simulink library "rst_controller_lib"  (Simulink 4.00)
undefined symbols (not defined in the file or in its folder): motor_1, parameters, rst_controller_sysCallback
settings Model: LastModifiedBy=Nick Donaldson

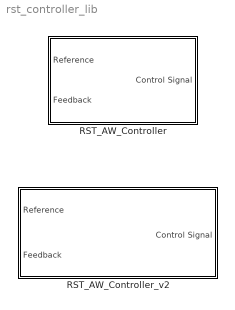
== system rst_controller_lib ==
  RST_AW_Controller : Subsystem  mask(RST Controller Design){Get_Controller_file=on, controll_fname='GLA_BEN_04_02_23_motorSim_1', R=motor_1.Controller_Design_1.rst_ctrl.R, S=motor_1.Controller_Design_1.rst_ctrl.S, T=motor_1.Controller_Design_1.rst_ctrl.T, Aaw=motor_1.Controller_Design_1.rst_ctrl.Aaw, Aaw_R=motor_1.Controller_Design_1.rst_ctrl.Aaw_R, out_limit=parameters.motor_controller.saturation_limit, sT=parameters.motor_controller.sample_time}
      mask prompts: Get_Controller_file "Get Controller from File"; controll_fname "Controller file name"; Aaw_R "Aaw - R"; out_limit "Output limitations"; sT "Sample time"
      mask help: Design of a controller that takes the form R*u = T*ref - S*output
      mask init:
      | if Get_Controller_file
      |    ctr_data = load(['Controllers\', controll_fname]);
      |    R = ctr_data.controllerData.rst.rst_ctrl.R;
      |    S = ctr_data.controllerData.rst.rst_ctrl.S;
      |    T = ctr_data.controllerData.rst.rst_ctrl.T;
      |    Aaw = ctr_data.controllerData.rst.rst_ctrl.Aaw;
      |    Aaw_R = ctr_data.controllerData.rst.rst_ctrl.Aaw_R;
      | end
      settings: RTWFcnNameOpts=Auto  RTWFileNameOpts=Auto
      mask CallbackString:
      | mv = get_param(gcb, 'MaskValues');
      |  if strcmp(mv{1}, 'on') a = 'on'; b = 'off';
      |  else a = 'off'; b = 'on';
      |  end;
      |  me = get_param(gcb, 'MaskEnables');
      |  me{2} = a;
      |  me{3} = b;
      |  me{4} = b;
      |  me{5} = b;
      |  me{6} = b;
      |  me{7} = b;
      |  set_param(gcb, 'MaskEnables', me);
      | ||||||||
      mask Display:
      | port_label('input', 1, 'Ref');
      | port_label('input', 2, 'Feedbk');
      | 
      | plot([0.01 0.05 0.01].*0.6+0.3, [0.82 0.8 0.78]);
      | plot([0.95 0.99 0.95].*0.6+0.3, [0.82 0.8 0.78]);
      | plot([0.52 0.48 0.52].*0.6+0.3, [0.22 0.2 0.18]);
      | 
      | plot([0.05 0.15 0.25; 0.25 0.15 0.35].*0.6+0.3, [0.8 0.2 0.6; 0.8 0.8 0.3]);
      | plot((0.25+0.1.*sin([0:pi/90:pi])).*0.6+0.3,0.7+0.1.*cos([0:pi/90:pi]));
      | plot([0.18 0.18; 0.18 0.25].*0.6+0.3, [0.3 0.75; 0.75 0.75]);
      | 
      | plot([0.35 0.5; 0.5 0.99].*0.6+0.3, [0.3 0.8; 0.3 0.8]);
      | plot((0.5+0.1.*sin([-pi:pi/90:0])).*0.6+0.3,0.7+0.1.*cos([0:pi/90:pi]));
      | plot((0.5+0.1.*sin([0:pi/90:pi])).*0.6+0.3,0.45+0.15.*cos([0:pi/90:pi]));
      | plot((0.5+0.07.*sin([-pi:pi/90:0])).*0.6+0.3,0.7+0.05.*cos([0:pi/90:pi]));
      | plot([0.5 0.6].*0.6+0.3, [0.75 0.75]);
      | 
      | plot([0.75 0.75; 0.75 0.15].*0.6+0.3, [0.8 0.2; 0.2 0.2]);
      | plot([0.85 0.78; 0.78 0.78].*0.6+0.3, [0.75 0.75; 0.75 0.3]);
      | 
      | text(0.5, 0.1, 'Anti-reset Control', 'VerticalAlignment', 'middle', 'HorizontalAlignment', 'center');
  RST_AW_Controller_v2 : Subsystem  InitFcn=rst_controller_sysCallback(gcb, 2);  mask(RST Controller Design){out_limit=[0 100]}
      mask prompts: out_limit "Output limitations"
      mask help: Design of a controller that takes the form R*u = T*ref - S*output
      mask init:
      | ctr_filename = get_param(gcb, 'UserData');
      | if isempty(ctr_filename)
      |    ctr_filename_disp = '? ? ? ? ?';
      | else
      |    [p n e v] = fileparts(ctr_filename);
      |    ctr_filename_disp = [n, e];
      |    ctr_data = load(ctr_filename, '-mat');
      |    R = ctr_data.controllerData.rst.rst_ctrl.R;
      |    S = ctr_data.controllerData.rst.rst_ctrl.S;
      |    T = ctr_data.controllerData.rst.rst_ctrl.T;
      |    Aaw = ctr_data.controllerData.rst.rst_ctrl.Aaw;
      |    Aaw_R = ctr_data.controllerData.rst.rst_ctrl.Aaw_R;
      |    sT = ctr_data.controllerData.rst.rst_ctrl.Ts;
      | end
      settings: OpenFcn=rst_controller_sysCallback(gcb, 11);  RTWFcnNameOpts=Auto  RTWFileNameOpts=Auto
      mask Display:
      | port_label('input', 1, 'Ref');
      | port_label('input', 2, 'Feedbk');
      | 
      | plot([0.01 0.05 0.01].*0.6+0.3, [0.82 0.8 0.78]);
      | plot([0.95 0.99 0.95].*0.6+0.3, [0.82 0.8 0.78]);
      | plot([0.52 0.48 0.52].*0.6+0.3, [0.22 0.2 0.18]);
      | 
      | plot([0.05 0.15 0.25; 0.25 0.15 0.35].*0.6+0.3, [0.8 0.2 0.6; 0.8 0.8 0.3]);
      | plot((0.25+0.1.*sin([0:pi/90:pi])).*0.6+0.3,0.7+0.1.*cos([0:pi/90:pi]));
      | plot([0.18 0.18; 0.18 0.25].*0.6+0.3, [0.3 0.75; 0.75 0.75]);
      | 
      | plot([0.35 0.5; 0.5 0.99].*0.6+0.3, [0.3 0.8; 0.3 0.8]);
      | plot((0.5+0.1.*sin([-pi:pi/90:0])).*0.6+0.3,0.7+0.1.*cos([0:pi/90:pi]));
      | plot((0.5+0.1.*sin([0:pi/90:pi])).*0.6+0.3,0.45+0.15.*cos([0:pi/90:pi]));
      | plot((0.5+0.07.*sin([-pi:pi/90:0])).*0.6+0.3,0.7+0.05.*cos([0:pi/90:pi]));
      | plot([0.5 0.6].*0.6+0.3, [0.75 0.75]);
      | 
      | plot([0.75 0.75; 0.75 0.15].*0.6+0.3, [0.8 0.2; 0.2 0.2]);
      | plot([0.85 0.78; 0.78 0.78].*0.6+0.3, [0.75 0.75; 0.75 0.3]);
      | 
      | text(0.5, 0.9, ctr_filename_disp, 'VerticalAlignment', 'middle', 'HorizontalAlignment', 'center');
      | text(0.5, 0.1, 'Anti-reset Control', 'VerticalAlignment', 'middle', 'HorizontalAlignment', 'center');

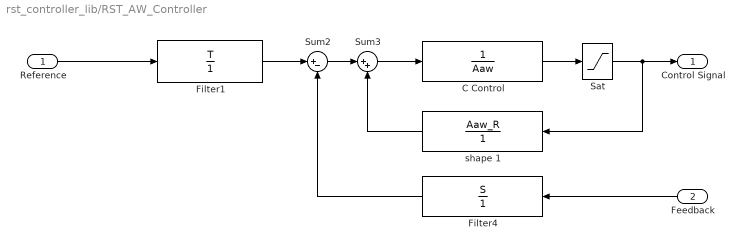
== system rst_controller_lib/RST_AW_Controller ==
  Reference : Inport  Port=1  LatchInput=off
  Feedback : Inport  Orientation=left  Port=2  LatchInput=off
  C Control : DiscreteFilter  Numerator=1  Denominator=Aaw  SampleTime=sT  Realization=auto
      settings: RTWStateStorageClass=Auto
  Filter1 : DiscreteFilter  Numerator=T  Denominator=1  SampleTime=sT  Realization=auto
      settings: RTWStateStorageClass=Auto
  Filter4 : DiscreteFilter  Orientation=left  Numerator=S  Denominator=1  SampleTime=sT  Realization=auto
      settings: RTWStateStorageClass=Auto
  Sat : Saturate  UpperLimit=out_limit(2)  LowerLimit=out_limit(1)  LinearizeAsGain=on
  Sum2 : Sum  Inputs=|+-  SaturateOnIntegerOverflow=on
  Sum3 : Sum  Inputs=|++  SaturateOnIntegerOverflow=on
  shape 1 : DiscreteFilter  Orientation=left  Numerator=Aaw_R  Denominator=1  SampleTime=sT  Realization=auto
      settings: RTWStateStorageClass=Auto
  Control Signal : Outport  Port=1
  wires:
  Filter4/1 -> Sum2/2
  Sum2/1 -> Sum3/1
  Filter1/1 -> Sum2/1
  Feedback/1 -> Filter4/1
  shape 1/1 -> Sum3/2
  C Control/1 -> Sat/1
  Sum3/1 -> C Control/1
  Sat/1 -> shape 1/1, Control Signal/1
  Reference/1 -> Filter1/1

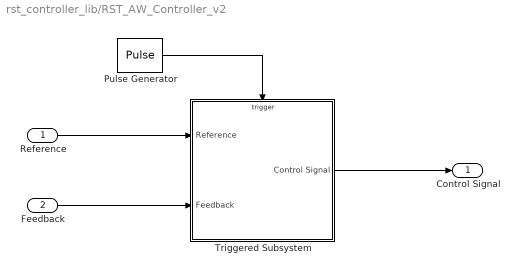
== system rst_controller_lib/RST_AW_Controller_v2 ==
  Reference : Inport  Port=1  LatchInput=off
  Feedback : Inport  Port=2  LatchInput=off
  Pulse Generator : DiscretePulseGenerator  PulseType=Time-based  Amplitude=1  Period=2*sT  PulseWidth=50  PhaseDelay=0  SampleTime=1
  Triggered Subsystem : Subsystem  TreatAsAtomicUnit=on
      settings: RTWFcnNameOpts=Auto  RTWFileNameOpts=Auto
  Control Signal : Outport  Port=1
  wires:
  Pulse Generator/1 -> Triggered Subsystem/Trigger
  Triggered Subsystem/1(Control Signal) -> Control Signal/1
  Feedback/1 -> Triggered Subsystem/2(Feedback)
  Reference/1 -> Triggered Subsystem/1(Reference)

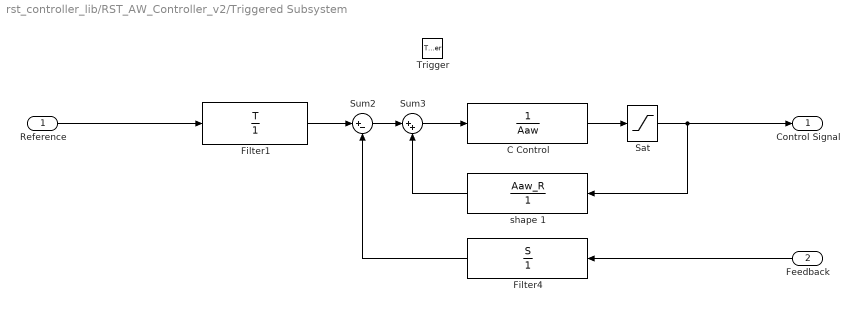
== system rst_controller_lib/RST_AW_Controller_v2/Triggered Subsystem ==
  Reference : Inport  Port=1  LatchInput=off
  Feedback : Inport  Orientation=left  Port=2  LatchInput=off
  Trigger : TriggerPort  TriggerType=either  OutputDataType=auto
  C Control : DiscreteFilter  Numerator=1  Denominator=Aaw  SampleTime=-1  Realization=auto
      settings: RTWStateStorageClass=Auto
  Filter1 : DiscreteFilter  Numerator=T  Denominator=1  SampleTime=-1  Realization=auto
      settings: RTWStateStorageClass=Auto
  Filter4 : DiscreteFilter  Orientation=left  Numerator=S  Denominator=1  SampleTime=-1  Realization=auto
      settings: RTWStateStorageClass=Auto
  Sat : Saturate  UpperLimit=out_limit(2)  LowerLimit=out_limit(1)  LinearizeAsGain=on
  Sum2 : Sum  Inputs=|+-  SaturateOnIntegerOverflow=on
  Sum3 : Sum  Inputs=|++  SaturateOnIntegerOverflow=on
  shape 1 : DiscreteFilter  Orientation=left  Numerator=Aaw_R  Denominator=1  SampleTime=-1  Realization=auto
      settings: RTWStateStorageClass=Auto
  Control Signal : Outport  Port=1
  wires:
  Reference/1 -> Filter1/1
  Sat/1 -> shape 1/1, Control Signal/1
  Sum3/1 -> C Control/1
  C Control/1 -> Sat/1
  shape 1/1 -> Sum3/2
  Feedback/1 -> Filter4/1
  Filter1/1 -> Sum2/1
  Sum2/1 -> Sum3/1
  Filter4/1 -> Sum2/2
